simulink model "Simple_4Quad_payload_09_2017a"  (R2018b)
settings: Solver=ode45  StartTime=0.0  StopTime=40  RelTol=1e-3
InitFcn:
  | Simple_4Quad_payload_09_const
values from neighbouring files (symbols this model uses):
  All_rho = [d1 0 0 ... (first row only)    [Colab_4Quad_model_01_const.m]    (also in Colab_4Quad_model_02_const.m; Simple_4Quad_payload_04_const.m; Simple_4Quad_payload_05_const.m; Simple_4Quad_payload_06_const.m)
  alpha_chatt = 0.1    [Simple_4Quad_payload_09_const.m]    (also in Simple_4Quad_payload_10_const.m = 0.001; Simple_4Quad_payload_11_const.m = 0.01; Simple_4Quad_payload_12_const.m = 0.01)
  alphaTF = 0.1    [Simple_4Quad_payload_08_const.m]    (also in Simple_4Quad_payload_09_const.m = 0.5; Simple_4Quad_payload_10_const.m = 1; Simple_4Quad_payload_11_const.m = 0.5; Simple_4Quad_payload_12_const.m = 10)
  B_ob = [zeros(3);eye(3)]    [Simple_4Quad_payload_04_const.m]    (also in Simple_4Quad_payload_05_const.m; Simple_4Quad_payload_06_const.m; Simple_4Quad_payload_07_const.m; Simple_4Quad_payload_08_const.m)
  BBT_inv = ((B'*B)^(-1))*B'    [Simple_2Quad_payload_03_const.m]    (also in Simple_4Quad_payload_04_const.m = ((BR'*BR)^(-1))*BR'; Simple_4Quad_payload_05_const.m = ((BR'*BR)^(-1))*BR'; Simple_4Quad_payload_06_const.m = ((BR'*BR)^(-1))*BR'; Simple_4Quad_payload_07_const.m = ((BR'*BR)^(-1))*BR')
  BR = 1e0*eye(n)    [Simple_4Quad_payload_04_const.m]    (also in Simple_4Quad_payload_05_const.m; Simple_4Quad_payload_06_const.m; Simple_4Quad_payload_07_const.m; Simple_4Quad_payload_08_const.m)
  C_ob = [eye(3) zeros(3)]    [Simple_4Quad_payload_04_const.m]    (also in Simple_4Quad_payload_05_const.m; Simple_4Quad_payload_06_const.m; Simple_4Quad_payload_07_const.m; Simple_4Quad_payload_08_const.m)
  d1 = 0.25    [Colab_4Quad_model_01_const.m]    (also in Colab_4Quad_model_02_const.m = 0.5; Simple_4Quad_payload_01_const.m = 1; Simple_4Quad_payload_02_const.m = 1; Simple_4Quad_payload_03_const.m = 1)
  d2 = 0.25    [Colab_4Quad_model_01_const.m]    (also in Colab_4Quad_model_02_const.m = 0.5; Simple_4Quad_payload_01_const.m = 1; Simple_4Quad_payload_02_const.m = 1; Simple_4Quad_payload_03_const.m = 1)
  Des_rel_dist = 2    [Simple_4Quad_payload_01_const.m]    (also in Simple_4Quad_payload_02_const.m = 4; Simple_4Quad_payload_03_const.m = 4; Simple_4Quad_payload_04_const.m; Simple_4Quad_payload_05_const.m)
  g = 9.81    [Colab_4Quad_model_01_const.m]    (also in Colab_4Quad_model_02_const.m; Simple_2Quad_payload_01_const.m; Simple_2Quad_payload_02_const.m; Simple_2Quad_payload_03_const.m)
  gamma_0 = 1e-0*diag([1e-3;1e-0])    [Simple_2Quad_payload_03_const.m]    (also in Simple_4Quad_payload_04_const.m = 1e-0*diag([1e-6*ones(3,1);1e-0*ones(3,1)]); Simple_4Quad_payload_05_const.m = 1e-1*diag([1e-6*ones(3,1);1e-0*ones(3,1)]); Simple_4Quad_payload_06_const.m = 1e-0*diag([1e-6*ones(3,1);1e-0*ones(3,1)]); Simple_4Quad_payload_07_const.m = 1e-0*diag([1e-6*ones(3,1);1e-0*ones(3,1)]))
  gamma_0L = 1e-0*diag([1e-6*ones(3,1);1e-0*ones(3,1)])    [Simple_4Quad_payload_08_const.m]    (also in Simple_4Quad_payload_09_const.m; Simple_4Quad_payload_10_const.m = 1e+0*diag([1e-3*ones(3,1);1e-3*ones(3,1)]); Simple_4Quad_payload_11_const.m = 1e+0*diag([1e-3*ones(3,1);1e-3*ones(3,1)]); Simple_4Quad_payload_12_const.m = 1e+2*diag(1e-4*ones(3,1)))
  gamma_0v = 1e-0*diag([1e-0*ones(3,1);1e-0*ones(3,1)])    [Simple_4Quad_payload_08_const.m]    (also in Simple_4Quad_payload_09_const.m = 1e-0*diag([1e-6*ones(3,1);1e-6*ones(3,1)]); Simple_4Quad_payload_10_const.m = 1e+0*diag(1e-0*ones(3,1)); Simple_4Quad_payload_11_const.m = 1e+0*diag(1e-0*ones(3,1)); Simple_4Quad_payload_12_const.m = 1e+3*diag(1e-0*ones(3,1)))
  gamma_1 = 1e+2*diag([1e-3;1e-0])    [Simple_2Quad_payload_03_const.m]    (also in Simple_4Quad_payload_04_const.m = 1e+2*diag([1e-6*ones(3,1);1e-0*ones(3,1)]); Simple_4Quad_payload_05_const.m = 1e+2*diag([1e-6*ones(3,1);1e-0*ones(3,1)]); Simple_4Quad_payload_06_const.m = 1e+3*diag([1e-6*ones(3,1);1e-0*ones(3,1)]); Simple_4Quad_payload_07_const.m = 1e+3*diag([1e-6*ones(3,1);1e-0*ones(3,1)]))
  gamma_1L = 1e+3*diag([1e-6*ones(3,1);1e-0*ones(3,1)])    [Simple_4Quad_payload_08_const.m]    (also in Simple_4Quad_payload_09_const.m = 1e+2*diag([1e-6*ones(3,1);1e-0*ones(3,1)]); Simple_4Quad_payload_10_const.m = 1e+1*diag([1e-3*ones(3,1);1e-3*ones(3,1)]); Simple_4Quad_payload_11_const.m = 1e+0*diag([1e-3*ones(3,1);1e-3*ones(3,1)]); Simple_4Quad_payload_12_const.m = 1e+2*diag(1e-4*ones(3,1)))
  gamma_1v = 1e+3*diag([1e-0*ones(3,1);1e-0*ones(3,1)])    [Simple_4Quad_payload_08_const.m]    (also in Simple_4Quad_payload_09_const.m = 1e+2*diag([1e-6*ones(3,1);1e-6*ones(3,1)]); Simple_4Quad_payload_10_const.m = 1e+0*diag(1e-0*ones(3,1)); Simple_4Quad_payload_11_const.m = 1e+0*diag(1e-0*ones(3,1)); Simple_4Quad_payload_12_const.m = 1e+3*diag(1e-0*ones(3,1)))
  Ix = 0.166667    [Colab_4Quad_model_01_const.m]    (also in Colab_4Quad_model_02_const.m = 0.02; Simple_4Quad_payload_01_const.m = 1; Simple_4Quad_payload_02_const.m = 1; Simple_4Quad_payload_03_const.m = 1)
  Iy = 0.166667    [Colab_4Quad_model_01_const.m]    (also in Colab_4Quad_model_02_const.m = 0.02; Simple_4Quad_payload_01_const.m = 1; Simple_4Quad_payload_02_const.m = 1; Simple_4Quad_payload_03_const.m = 1)
  Iz = 0.166667    [Colab_4Quad_model_01_const.m]    (also in Colab_4Quad_model_02_const.m = 0.02; Simple_4Quad_payload_01_const.m = 1; Simple_4Quad_payload_02_const.m = 1; Simple_4Quad_payload_03_const.m = 1)
  Jo = diag([Ix;Iy;Iz])    [Colab_4Quad_model_01_const.m]    (also in Colab_4Quad_model_02_const.m; Simple_4Quad_payload_04_const.m; Simple_4Quad_payload_05_const.m; Simple_4Quad_payload_06_const.m)
  Jq = diag([0.0291 0.0291 0.0552])    [Colab_4Quad_model_01_const.m]    (also in Colab_4Quad_model_02_const.m = diag([0.03 0.03 0.06]); Simple_4Quad_payload_03_const.m = 1.2416e-3 * diag([1 1 2]); Simple_4Quad_payload_04_const.m = 1 * diag([1 1 2]); Simple_4Quad_payload_05_const.m = 1 * diag([1 1 2]))
  k1 = 1    [Simple_2Quad_payload_03_const.m]    (also in Simple_4Quad_payload_04_const.m; Simple_4Quad_payload_05_const.m; Simple_4Quad_payload_06_const.m; Simple_4Quad_payload_07_const.m)
  k2 = 0.1    [Simple_2Quad_payload_03_const.m]    (also in Simple_4Quad_payload_04_const.m; Simple_4Quad_payload_05_const.m; Simple_4Quad_payload_06_const.m; Simple_4Quad_payload_07_const.m)
  l = 3.1819    [Colab_4Quad_model_01_const.m]    (also in Colab_4Quad_model_02_const.m = 3; Simple_2Quad_payload_04_const.m = 1; Simple_4Quad_payload_01_const.m = 1; Simple_4Quad_payload_02_const.m = 2)
  m = 1.5    [Colab_4Quad_model_01_const.m]    (also in Colab_4Quad_model_02_const.m; Simple_2Quad_payload_04_const.m = 1; Simple_4Quad_payload_01_const.m = 1; Simple_4Quad_payload_02_const.m = 1)
  M = 1.0    (= 1)    [Colab_4Quad_model_01_const.m]    (also in Colab_4Quad_model_02_const.m; Simple_2Quad_payload_01_const.m; Simple_2Quad_payload_02_const.m; Simple_2Quad_payload_03_const.m)
  n = 2    [Simple_2Quad_payload_03_const.m]    (also in Simple_4Quad_payload_03_const.m = 6; Simple_4Quad_payload_04_const.m = 6; Simple_4Quad_payload_05_const.m = 6; Simple_4Quad_payload_06_const.m = 6)
  noise_var_Omegao = 0e-6    (= 0)    [Simple_4Quad_payload_07_const.m]    (also in Simple_4Quad_payload_08_const.m; Simple_4Quad_payload_09_const.m; Simple_4Quad_payload_10_const.m; Simple_4Quad_payload_11_const.m)
  noise_var_RelAcc = 0e-6    (= 0)    [Simple_4Quad_payload_07_const.m]    (also in Simple_4Quad_payload_08_const.m; Simple_4Quad_payload_09_const.m; Simple_4Quad_payload_10_const.m; Simple_4Quad_payload_11_const.m)
  noise_var_RelPos = 0e-6    (= 0)    [Simple_4Quad_payload_07_const.m]    (also in Simple_4Quad_payload_08_const.m; Simple_4Quad_payload_09_const.m; Simple_4Quad_payload_10_const.m; Simple_4Quad_payload_11_const.m)
  Q_ob = var_u_ob * eye(6)    [Simple_4Quad_payload_04_const.m]    (also in Simple_4Quad_payload_05_const.m; Simple_4Quad_payload_06_const.m; Simple_4Quad_payload_07_const.m; Simple_4Quad_payload_08_const.m)
  QL = 1e-0*eye(n)    [Simple_4Quad_payload_08_const.m]    (also in Simple_4Quad_payload_09_const.m; Simple_4Quad_payload_10_const.m; Simple_4Quad_payload_11_const.m = 1e-2*eye(n); Simple_4Quad_payload_12_const.m = 1e-0*eye(np))
  QR = 1e-0*eye(n)    [Simple_4Quad_payload_04_const.m]    (also in Simple_4Quad_payload_05_const.m = 1e-1*eye(n); Simple_4Quad_payload_06_const.m; Simple_4Quad_payload_07_const.m; Simple_4Quad_payload_08_const.m)
  Qv = 1e-0*eye(n)    [Simple_4Quad_payload_08_const.m]    (also in Simple_4Quad_payload_09_const.m; Simple_4Quad_payload_10_const.m = 1e-0*eye(np); Simple_4Quad_payload_11_const.m = 1e-2*eye(np); Simple_4Quad_payload_12_const.m = 1e-0*eye(np))
  R = 1e+0*eye(n)    [Simple_2Quad_payload_03_const.m]    (also in Simple_4Quad_payload_04_const.m = 1e+0*eye(m); Simple_4Quad_payload_05_const.m = 1e+0*eye(m); Simple_4Quad_payload_06_const.m; Simple_4Quad_payload_07_const.m)
  R_ob = var_y_ob * eye(3)    [Simple_4Quad_payload_04_const.m]    (also in Simple_4Quad_payload_05_const.m; Simple_4Quad_payload_06_const.m; Simple_4Quad_payload_07_const.m; Simple_4Quad_payload_08_const.m)
  rho_0 = 1e-0    (= 1)    [Simple_2Quad_payload_03_const.m]    (also in Simple_4Quad_payload_04_const.m; Simple_4Quad_payload_05_const.m = 0.1; Simple_4Quad_payload_06_const.m; Simple_4Quad_payload_07_const.m)
  rho_0L = 1e-0    (= 1)    [Simple_4Quad_payload_08_const.m]    (also in Simple_4Quad_payload_09_const.m; Simple_4Quad_payload_10_const.m; Simple_4Quad_payload_11_const.m; Simple_4Quad_payload_12_const.m)
  rho_0v = 1e-1    (= 0.1)    [Simple_4Quad_payload_08_const.m]    (also in Simple_4Quad_payload_09_const.m = 1; Simple_4Quad_payload_10_const.m = 1; Simple_4Quad_payload_11_const.m = 1; Simple_4Quad_payload_12_const.m = 1)
  rho_1 = 1e-0    (= 1)    [Simple_2Quad_payload_03_const.m]    (also in Simple_4Quad_payload_04_const.m; Simple_4Quad_payload_05_const.m; Simple_4Quad_payload_06_const.m; Simple_4Quad_payload_07_const.m)
  rho_1L = 1e-0    (= 1)    [Simple_4Quad_payload_08_const.m]    (also in Simple_4Quad_payload_09_const.m; Simple_4Quad_payload_10_const.m; Simple_4Quad_payload_11_const.m; Simple_4Quad_payload_12_const.m)
  rho_1v = 1e-0    (= 1)    [Simple_4Quad_payload_08_const.m]    (also in Simple_4Quad_payload_09_const.m; Simple_4Quad_payload_10_const.m; Simple_4Quad_payload_11_const.m; Simple_4Quad_payload_12_const.m)
libraries: simulink x1
(part 1 of 4)
settings Model: Creator=ali  LastModifiedBy=asafae
settings SolverCC: ZeroCrossAlgorithm=Adaptive
settings DebuggingCC: IgnoredZcDiagnostic=none
settings CodeAppCC: StateflowObjectComments=on

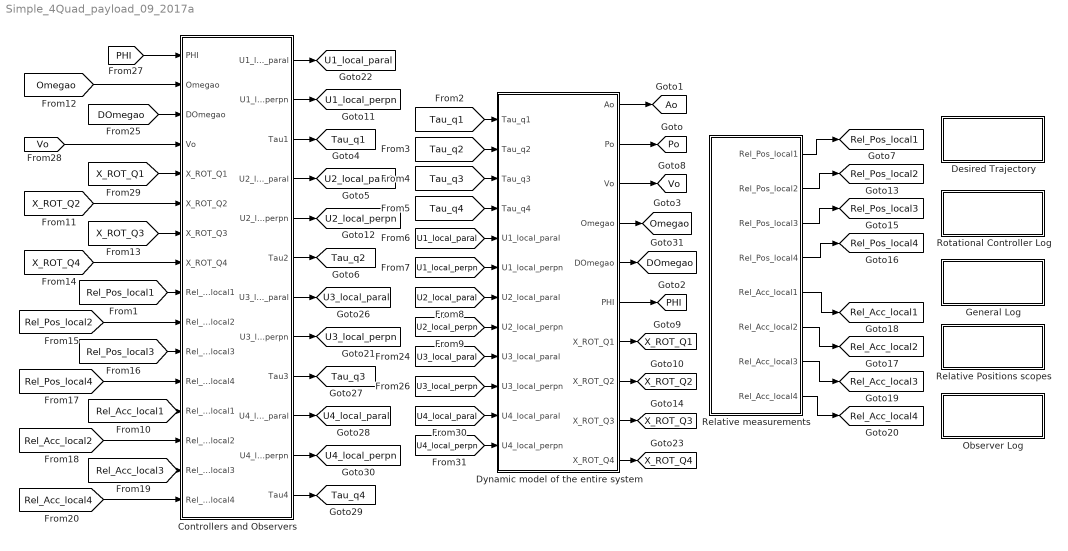
== system Simple_4Quad_payload_09_2017a ==
  Controllers and Observers : Subsystem
  Desired Trajectory : Subsystem
  Dynamic model of the entire system : Subsystem
  General Log : Subsystem
  Observer Log : Subsystem
  Relative Positions scopes : Subsystem
  Relative measurements : Subsystem
  Rotational Controller Log : Subsystem
  tag scope: Ao=global, DOmegao=global, Omegao=global, PHI=global, Po=global, Rel_Acc_local1=global, Rel_Acc_local2=global, Rel_Acc_local3=global, Rel_Acc_local4=global, Rel_Pos_local1=global, Rel_Pos_local2=global, Rel_Pos_local3=global, Rel_Pos_local4=global, Tau_q1=global, Tau_q2=global, Tau_q3=global, Tau_q4=global, U1_local_paral=global, U1_local_perpn=global, U2_local_paral=global, U2_local_perpn=global, U3_local_paral=global, U3_local_perpn=global, U4_local_paral=global, U4_local_perpn=global, Vo=global, X_ROT_Q1=global, X_ROT_Q2=global, X_ROT_Q3=global, X_ROT_Q4=global
  wires:
  [Tau_q1] -> Dynamic model of the entire system/1(Tau_q1)
  [Tau_q2] -> Dynamic model of the entire system/2(Tau_q2)
  [Tau_q3] -> Dynamic model of the entire system/3(Tau_q3)
  [Tau_q4] -> Dynamic model of the entire system/4(Tau_q4)
  [U1_local_paral] -> Dynamic model of the entire system/5(U1_local_paral)
  [U1_local_perpn] -> Dynamic model of the entire system/6(U1_local_perpn)
  Dynamic model of the entire system/6(PHI) -> [PHI]
  Dynamic model of the entire system/4(Omegao) -> [Omegao]
  Dynamic model of the entire system/1(Ao) -> [Ao]
  Dynamic model of the entire system/2(Po) -> [Po]
  Dynamic model of the entire system/5(DOmegao) -> [DOmegao]
  Dynamic model of the entire system/7(X_ROT_Q1) -> [X_ROT_Q1]
  Dynamic model of the entire system/8(X_ROT_Q2) -> [X_ROT_Q2]
  Dynamic model of the entire system/9(X_ROT_Q3) -> [X_ROT_Q3]
  Controllers and Observers/1(U1_local_paral) -> [U1_local_paral]
  Controllers and Observers/3(Tau1) -> [Tau_q1]
  Controllers and Observers/4(U2_local_paral) -> [U2_local_paral]
  Controllers and Observers/6(Tau2) -> [Tau_q2]
  Controllers and Observers/12(Tau4) -> [Tau_q4]
  Controllers and Observers/10(U4_local_paral) -> [U4_local_paral]
  Controllers and Observers/9(Tau3) -> [Tau_q3]
  Controllers and Observers/7(U3_local_paral) -> [U3_local_paral]
  [Omegao] -> Controllers and Observers/2(Omegao)
  [DOmegao] -> Controllers and Observers/3(DOmegao)
  [X_ROT_Q1] -> Controllers and Observers/5(X_ROT_Q1)
  [X_ROT_Q2] -> Controllers and Observers/6(X_ROT_Q2)
  [X_ROT_Q3] -> Controllers and Observers/7(X_ROT_Q3)
  [X_ROT_Q4] -> Controllers and Observers/8(X_ROT_Q4)
  [Rel_Pos_local1] -> Controllers and Observers/9(Rel_Pos_local1)
  [Rel_Pos_local2] -> Controllers and Observers/10(Rel_Pos_local2)
  [Rel_Pos_local3] -> Controllers and Observers/11(Rel_Pos_local3)
  [Rel_Pos_local4] -> Controllers and Observers/12(Rel_Pos_local4)
  [Rel_Acc_local1] -> Controllers and Observers/13(Rel_Acc_local1)
  [Rel_Acc_local2] -> Controllers and Observers/14(Rel_Acc_local2)
  [Rel_Acc_local3] -> Controllers and Observers/15(Rel_Acc_local3)
  [Rel_Acc_local4] -> Controllers and Observers/16(Rel_Acc_local4)
  Relative measurements/1(Rel_Pos_local1) -> [Rel_Pos_local1]
  Relative measurements/2(Rel_Pos_local2) -> [Rel_Pos_local2]
  Relative measurements/3(Rel_Pos_local3) -> [Rel_Pos_local3]
  Relative measurements/4(Rel_Pos_local4) -> [Rel_Pos_local4]
  Relative measurements/5(Rel_Acc_local1) -> [Rel_Acc_local1]
  Relative measurements/6(Rel_Acc_local2) -> [Rel_Acc_local2]
  Relative measurements/7(Rel_Acc_local3) -> [Rel_Acc_local3]
  Relative measurements/8(Rel_Acc_local4) -> [Rel_Acc_local4]
  Dynamic model of the entire system/3(Vo) -> [Vo]
  [Vo] -> Controllers and Observers/4(Vo)
  [PHI] -> Controllers and Observers/1(PHI)
  Controllers and Observers/2(U1_local_perpn) -> [U1_local_perpn]
  Controllers and Observers/5(U2_local_perpn) -> [U2_local_perpn]
  Controllers and Observers/8(U3_local_perpn) -> [U3_local_perpn]
  Controllers and Observers/11(U4_local_perpn) -> [U4_local_perpn]
  [U2_local_paral] -> Dynamic model of the entire system/7(U2_local_paral)
  [U2_local_perpn] -> Dynamic model of the entire system/8(U2_local_perpn)
  [U3_local_paral] -> Dynamic model of the entire system/9(U3_local_paral)
  [U4_local_paral] -> Dynamic model of the entire system/11(U4_local_paral)
  [U4_local_perpn] -> Dynamic model of the entire system/12(U4_local_perpn)
  [U3_local_perpn] -> Dynamic model of the entire system/10(U3_local_perpn)
  Dynamic model of the entire system/10(X_ROT_Q4) -> [X_ROT_Q4]

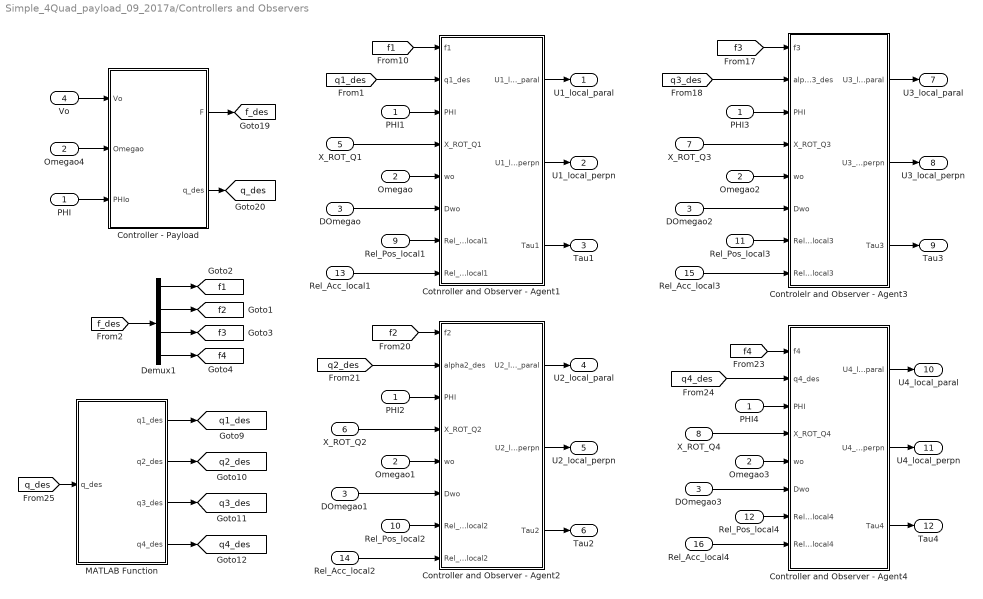
== system Simple_4Quad_payload_09_2017a/Controllers and Observers ==
  PHI : Inport
  Omegao : Inport  Port=2
  DOmegao : Inport  Port=3
  Vo : Inport  Port=4
  X_ROT_Q1 : Inport  Port=5
  X_ROT_Q2 : Inport  Port=6
  X_ROT_Q3 : Inport  Port=7
  X_ROT_Q4 : Inport  Port=8
  Rel_Pos_local1 : Inport  Port=9
  Rel_Pos_local2 : Inport  Port=10
  Rel_Pos_local3 : Inport  Port=11
  Rel_Pos_local4 : Inport  Port=12
  Rel_Acc_local1 : Inport  Port=13
  Rel_Acc_local2 : Inport  Port=14
  Rel_Acc_local3 : Inport  Port=15
  Rel_Acc_local4 : Inport  Port=16
  Controlelr and Observer - Agent3 : Subsystem
  Controller - Payload : Subsystem
  Controller and Observer - Agent2 : Subsystem
  Controller and Observer - Agent4 : Subsystem
  "Cotnroller and Observer - Agent1 " : Subsystem
  DOmegao1 : InportShadow  Port=3
  DOmegao2 : InportShadow  Port=3
  DOmegao3 : InportShadow  Port=3
  Demux1 : Demux
  MATLAB Function : MATLAB Function  TreatAsAtomicUnit=on
  Omegao{1..4} (4 alike) : InportShadow  Port=2
  PHI{1..4} (4 alike) : InportShadow
  U1_local_paral : Outport
  U1_local_perpn : Outport  Port=2
  Tau1 : Outport  Port=3
  U2_local_paral : Outport  Port=4
  U2_local_perpn : Outport  Port=5
  Tau2 : Outport  Port=6
  U3_local_paral : Outport  Port=7
  U3_local_perpn : Outport  Port=8
  Tau3 : Outport  Port=9
  U4_local_paral : Outport  Port=10
  U4_local_perpn : Outport  Port=11
  Tau4 : Outport  Port=12
  tag scope: f1=global, f2=global, f3=global, f4=global, f_des=global, q1_des=global, q2_des=global, q3_des=global, q4_des=global, q_des=global
  wires:
  Controller and Observer - Agent4/3(Tau4) -> Tau4/1
  Controller and Observer - Agent4/1(U4_local_paral) -> U4_local_paral/1
  Controlelr and Observer - Agent3/3(Tau3) -> Tau3/1
  Controlelr and Observer - Agent3/1(U3_local_paral) -> U3_local_paral/1
  Controller and Observer - Agent2/1(U2_local_paral) -> U2_local_paral/1
  "Cotnroller and Observer - Agent1 "/1(U1_local_paral) -> U1_local_paral/1
  Controller and Observer - Agent2/3(Tau2) -> Tau2/1
  X_ROT_Q1/1 -> "Cotnroller and Observer - Agent1 "/4(X_ROT_Q1)
  X_ROT_Q3/1 -> Controlelr and Observer - Agent3/4(X_ROT_Q3)
  X_ROT_Q4/1 -> Controller and Observer - Agent4/4(X_ROT_Q4)
  X_ROT_Q2/1 -> Controller and Observer - Agent2/4(X_ROT_Q2)
  "Cotnroller and Observer - Agent1 "/3(Tau1) -> Tau1/1
  [f1] -> "Cotnroller and Observer - Agent1 "/1(f1)
  Controller - Payload/2(q_des) -> [q_des]
  Vo/1 -> Controller - Payload/1(Vo)
  Omegao4/1 -> Controller - Payload/2(Omegao)
  PHI/1 -> Controller - Payload/3(PHIo)
  Controller - Payload/1(F) -> [f_des]
  Rel_Pos_local1/1 -> "Cotnroller and Observer - Agent1 "/7(Rel_Pos_local1)
  Rel_Acc_local1/1 -> "Cotnroller and Observer - Agent1 "/8(Rel_Acc_local1)
  Rel_Pos_local2/1 -> Controller and Observer - Agent2/7(Rel_Pos_local2)
  Rel_Acc_local2/1 -> Controller and Observer - Agent2/8(Rel_Acc_local2)
  Rel_Pos_local4/1 -> Controller and Observer - Agent4/7(Rel_Pos_local4)
  Rel_Acc_local4/1 -> Controller and Observer - Agent4/8(Rel_Acc_local4)
  Rel_Pos_local3/1 -> Controlelr and Observer - Agent3/7(Rel_Pos_local3)
  Rel_Acc_local3/1 -> Controlelr and Observer - Agent3/8(Rel_Acc_local3)
  [f3] -> Controlelr and Observer - Agent3/1(f3)
  [q3_des] -> Controlelr and Observer - Agent3/2(alpha3_des)
  [f2] -> Controller and Observer - Agent2/1(f2)
  [q2_des] -> Controller and Observer - Agent2/2(alpha2_des)
  [f4] -> Controller and Observer - Agent4/1(f4)
  [q4_des] -> Controller and Observer - Agent4/2(q4_des)
  DOmegao/1 -> "Cotnroller and Observer - Agent1 "/6(Dwo)
  DOmegao1/1 -> Controller and Observer - Agent2/6(Dwo)
  DOmegao2/1 -> Controlelr and Observer - Agent3/6(Dwo)
  DOmegao3/1 -> Controller and Observer - Agent4/6(Dwo)
  Omegao/1 -> "Cotnroller and Observer - Agent1 "/5(wo)
  Omegao2/1 -> Controlelr and Observer - Agent3/5(wo)
  Omegao1/1 -> Controller and Observer - Agent2/5(wo)
  Omegao3/1 -> Controller and Observer - Agent4/5(wo)
  Demux1/4 -> [f4]
  Demux1/1 -> [f1]
  [f_des] -> Demux1/1
  Demux1/3 -> [f3]
  Demux1/2 -> [f2]
  PHI1/1 -> "Cotnroller and Observer - Agent1 "/3(PHI)
  PHI2/1 -> Controller and Observer - Agent2/3(PHI)
  PHI3/1 -> Controlelr and Observer - Agent3/3(PHI)
  PHI4/1 -> Controller and Observer - Agent4/3(PHI)
  [q_des] -> MATLAB Function/1(q_des)
  [q1_des] -> "Cotnroller and Observer - Agent1 "/2(q1_des)
  "Cotnroller and Observer - Agent1 "/2(U1_local_perpn) -> U1_local_perpn/1
  Controller and Observer - Agent2/2(U2_local_perpn) -> U2_local_perpn/1
  Controlelr and Observer - Agent3/2(U3_local_perpn) -> U3_local_perpn/1
  Controller and Observer - Agent4/2(U4_local_perpn) -> U4_local_perpn/1
  MATLAB Function/4(q4_des) -> [q4_des]
  MATLAB Function/3(q3_des) -> [q3_des]
  MATLAB Function/2(q2_des) -> [q2_des]
  MATLAB Function/1(q1_des) -> [q1_des]

== system Simple_4Quad_payload_09_2017a/Desired Trajectory ==
  Clock : Clock
  Constant1 : Constant  Value=[0;0;0]
  Constant2 : Constant  Value=[0;0;2]
  Constant3 : Constant  Value=[0.3;0.5;2]
  Gain : Gain  Gain=0.01
  Gain1 : Gain  Gain=0.02
  MATLAB Function : MATLAB Function  TreatAsAtomicUnit=on
  Mux3 : Mux  Inputs=3
  Subsystem : Subsystem
  Switch : Switch  Criteria=u2 > Threshold  Threshold=10
  Switch1 : Switch  Criteria=u2 > Threshold  Threshold=20
  tag scope: Desired_Track=global
  wires:
  Constant3/1 -> Switch1/1
  Gain/1 -> Mux3/1
  Constant1/1 -> Switch/3
  Gain1/1 -> Mux3/2
  Switch/1 -> Switch1/3
  Constant2/1 -> Switch/1
  Switch1/1 -> Subsystem/1(In1)
  Clock/1 -> Gain1/1, Switch1/2, Switch/2, MATLAB Function/1(t), Gain/1
  Subsystem/1(Out1) -> [Desired_Track]

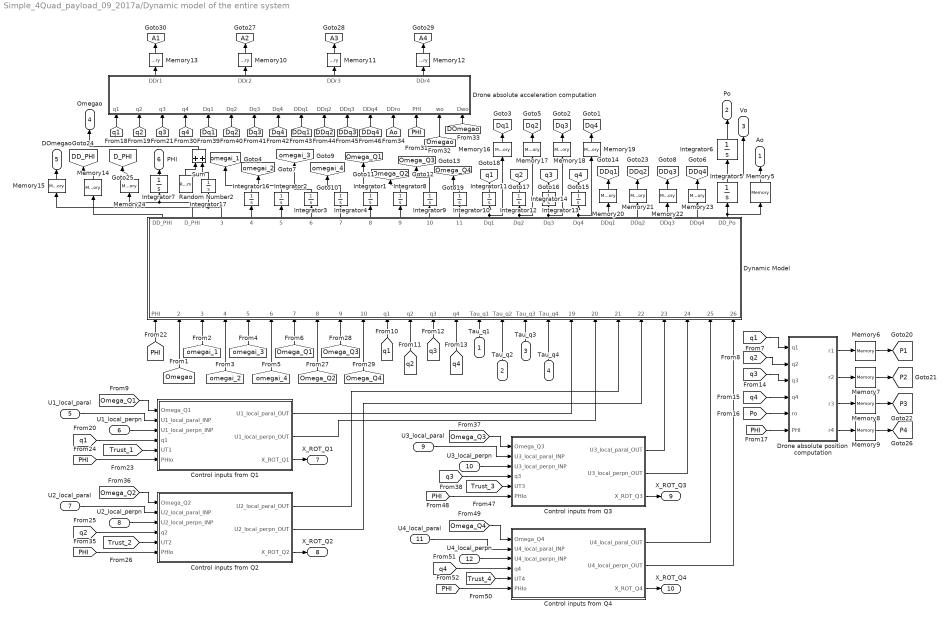
== system Simple_4Quad_payload_09_2017a/Dynamic model of the entire system ==
  Tau_q1 : Inport
  Tau_q2 : Inport  Port=2
  Tau_q3 : Inport  Port=3
  Tau_q4 : Inport  Port=4
  U1_local_paral : Inport  Port=5
  U1_local_perpn : Inport  Port=6
  U2_local_paral : Inport  Port=7
  U2_local_perpn : Inport  Port=8
  U3_local_paral : Inport  Port=9
  U3_local_perpn : Inport  Port=10
  U4_local_paral : Inport  Port=11
  U4_local_perpn : Inport  Port=12
  Control inputs from Q1 : Subsystem
  Control inputs from Q2 : Subsystem
  Control inputs from Q3 : Subsystem
  Control inputs from Q4 : Subsystem
  Drone absolute acceleration computation : MATLAB Function  TreatAsAtomicUnit=on
  Drone absolute position computation : MATLAB Function  TreatAsAtomicUnit=on
  "Dynamic Model " : MATLAB Function  TreatAsAtomicUnit=on
  Integrator{1..5,7..10,16..17} (11 alike) : Integrator  InitialCondition=zeros(3,1)
  Integrator{11..14} (4 alike) : Integrator  InitialCondition=[0;0;1]
  Integrator6 : Integrator  InitialCondition=[0;0;0]
  Memory{5,10..24} (16 alike) : Memory  InitialCondition=zeros(3,1)
  Memory6 : Memory  InitialCondition=[d1;0;l]
  Memory7 : Memory  InitialCondition=[-d1;0;l]
  Memory8 : Memory  InitialCondition=[0;d2;l]
  Memory9 : Memory  InitialCondition=[0;-d2;l]
  Random Number2 : RandomNumber  Variance=noise_var_Omegao  VectorParams1D=off
  Sum : Sum
  Ao : Outport
  Po : Outport  Port=2
  Vo : Outport  Port=3
  Omegao : Outport  Port=4
  DOmegao : Outport  Port=5
  PHI : Outport  Port=6
  X_ROT_Q1 : Outport  Port=7
  X_ROT_Q2 : Outport  Port=8
  X_ROT_Q3 : Outport  Port=9
  X_ROT_Q4 : Outport  Port=10
  tag scope: A1=global, A2=global, A3=global, A4=global, DD_PHI=global, DDq1=global, DDq2=global, DDq3=global, DDq4=global, D_PHI=global, Dq1=global, Dq2=global, Dq3=global, Dq4=global, Omega_Q1=global, Omega_Q2=global, Omega_Q3=global, Omega_Q4=global, P1=global, P2=global, P3=global, P4=global, omegai_1=global, omegai_2=global, omegai_3=global, omegai_4=global, q1=global, q2=global, q3=global, q4=global
  wires:
  Integrator5/1 -> Vo/1, Integrator6/1
  Integrator1/1 -> [Omega_Q1]
  Integrator2/1 -> [omegai_2]
  Integrator3/1 -> [omegai_3]
  Integrator6/1 -> Po/1
  Integrator4/1 -> [omegai_4]
  Memory5/1 -> Ao/1
  Integrator7/1 -> PHI/1
  "Dynamic Model "/20(DD_Po) -> Memory5/1, Integrator5/1
  "Dynamic Model "/2(D_PHI) -> Memory24/1, Integrator7/1
  "Dynamic Model "/1(DD_PHI) -> Memory14/1
  "Dynamic Model "/7(D_omegai_4) -> Integrator4/1
  "Dynamic Model "/6(D_omegai_3) -> Integrator3/1
  "Dynamic Model "/5(D_omegai_2) -> Integrator2/1
  "Dynamic Model "/4(D_omegai_1) -> Integrator16/1
  "Dynamic Model "/3(D_Omegao) -> Memory15/1, Integrator17/1
  Integrator16/1 -> [omegai_1]
  "Dynamic Model "/8(D_Omega_Q1) -> Integrator1/1
  "Dynamic Model "/9(D_Omega_Q2) -> Integrator8/1
  "Dynamic Model "/10(D_Omega_Q3) -> Integrator9/1
  "Dynamic Model "/11(D_Omega_Q4) -> Integrator10/1
  Integrator8/1 -> [Omega_Q2]
  Integrator10/1 -> [Omega_Q4]
  Integrator9/1 -> [Omega_Q3]
  "Dynamic Model "/12(Dq1) -> Memory16/1, Integrator11/1
  "Dynamic Model "/13(Dq2) -> Memory17/1, Integrator12/1
  "Dynamic Model "/14(Dq3) -> Memory18/1, Integrator13/1
  "Dynamic Model "/15(Dq4) -> Memory19/1, Integrator14/1
  Integrator14/1 -> [q4]
  Integrator13/1 -> [q3]
  Integrator12/1 -> [q2]
  Integrator11/1 -> [q1]
  [PHI] -> "Dynamic Model "/1(PHI)
  [Omegao] -> "Dynamic Model "/2(Omegao)
  [omegai_1] -> "Dynamic Model "/3(omegai1)
  [omegai_2] -> "Dynamic Model "/4(omegai2)
  [omegai_3] -> "Dynamic Model "/5(omegai3)
  [omegai_4] -> "Dynamic Model "/6(omegai4)
  [Omega_Q1] -> "Dynamic Model "/7(Omega_q1)
  [Omega_Q2] -> "Dynamic Model "/8(Omega_q2)
  [Omega_Q3] -> "Dynamic Model "/9(Omega_q3)
  [Omega_Q4] -> "Dynamic Model "/10(Omega_q4)
  [q1] -> "Dynamic Model "/11(q1)
  [q2] -> "Dynamic Model "/12(q2)
  [q3] -> "Dynamic Model "/13(q3)
  [q4] -> "Dynamic Model "/14(q4)
  Tau_q2/1 -> "Dynamic Model "/16(Tau_q2)
  Tau_q4/1 -> "Dynamic Model "/18(Tau_q4)
  Tau_q1/1 -> "Dynamic Model "/15(Tau_q1)
  Tau_q3/1 -> "Dynamic Model "/17(Tau_q3)
  Control inputs from Q1/1(U1_local_paral_OUT) -> "Dynamic Model "/19(U1_local_paral)
  [q1] -> Drone absolute position computation/1(q1)
  [q2] -> Drone absolute position computation/2(q2)
  [q3] -> Drone absolute position computation/3(q3)
  [q4] -> Drone absolute position computation/4(q4)
  [Po] -> Drone absolute position computation/5(ro)
  [PHI] -> Drone absolute position computation/6(PHI)
  Memory6/1 -> [P1]
  Memory8/1 -> [P3]
  Memory7/1 -> [P2]
  Memory9/1 -> [P4]
  Drone absolute position computation/4(r4) -> Memory9/1
  Drone absolute position computation/3(r3) -> Memory8/1
  Drone absolute position computation/2(r2) -> Memory7/1
  Drone absolute position computation/1(r1) -> Memory6/1
  [q1] -> Drone absolute acceleration computation/1(q1)
  [q2] -> Drone absolute acceleration computation/2(q2)
  [q3] -> Drone absolute acceleration computation/3(q3)
  [q4] -> Drone absolute acceleration computation/4(q4)
  [PHI] -> Drone absolute acceleration computation/14(PHI)
  [Omegao] -> Drone absolute acceleration computation/15(wo)
  Memory13/1 -> [A1]
  Drone absolute acceleration computation/1(DDr1) -> Memory13/1
  Memory10/1 -> [A2]
  Drone absolute acceleration computation/2(DDr2) -> Memory10/1
  Memory11/1 -> [A3]
  Drone absolute acceleration computation/3(DDr3) -> Memory11/1
  Memory12/1 -> [A4]
  Drone absolute acceleration computation/4(DDr4) -> Memory12/1
  Memory15/1 -> DOmegao/1
  [DOmegao] -> Drone absolute acceleration computation/16(Dwo)
  [Ao] -> Drone absolute acceleration computation/13(DDro)
  Memory19/1 -> [Dq4]
  Memory18/1 -> [Dq3]
  Memory16/1 -> [Dq1]
  Memory17/1 -> [Dq2]
  [Dq4] -> Drone absolute acceleration computation/8(Dq4)
  [Dq3] -> Drone absolute acceleration computation/7(Dq3)
  [Dq2] -> Drone absolute acceleration computation/6(Dq2)
  [Dq1] -> Drone absolute acceleration computation/5(Dq1)
  Memory21/1 -> [DDq2]
  Memory20/1 -> [DDq1]
  Memory22/1 -> [DDq3]
  Memory23/1 -> [DDq4]
  "Dynamic Model "/16(DDq1) -> Memory20/1
  "Dynamic Model "/17(DDq2) -> Memory21/1
  "Dynamic Model "/18(DDq3) -> Memory22/1
  "Dynamic Model "/19(DDq4) -> Memory23/1
  [DDq1] -> Drone absolute acceleration computation/9(DDq1)
  [DDq2] -> Drone absolute acceleration computation/10(DDq2)
  [DDq3] -> Drone absolute acceleration computation/11(DDq3)
  [DDq4] -> Drone absolute acceleration computation/12(DDq4)
  Memory24/1 -> [D_PHI]
  Control inputs from Q3/1(U3_local_paral_OUT) -> "Dynamic Model "/23(U3_local_paral)
  Control inputs from Q4/1(U4_local_paral_OUT) -> "Dynamic Model "/25(U4_local_paral)
  Control inputs from Q4/2(U4_local_perpn_OUT) -> "Dynamic Model "/26(U4_local_perpn)
  Control inputs from Q1/3(X_ROT_Q1) -> X_ROT_Q1/1
  [Omega_Q1] -> Control inputs from Q1/1(Omega_Q1)
  U1_local_paral/1 -> Control inputs from Q1/2(U1_local_paral_INP)
  U1_local_perpn/1 -> Control inputs from Q1/3(U1_local_perpn_INP)
  Control inputs from Q1/2(U1_local_perpn_OUT) -> "Dynamic Model "/20(U1_local_perpn)
  [q1] -> Control inputs from Q1/4(q1)
  [Trust_1] -> Control inputs from Q1/5(UT1)
  [PHI] -> Control inputs from Q1/6(PHIo)
  [PHI] -> Control inputs from Q2/6(PHIo)
  [Trust_2] -> Control inputs from Q2/5(UT2)
  [q2] -> Control inputs from Q2/4(q2)
  U2_local_perpn/1 -> Control inputs from Q2/3(U2_local_perpn_INP)
  U2_local_paral/1 -> Control inputs from Q2/2(U2_local_paral_INP)
  [Omega_Q2] -> Control inputs from Q2/1(Omega_Q2)
  Control inputs from Q2/3(X_ROT_Q2) -> X_ROT_Q2/1
  Control inputs from Q2/1(U2_local_paral_OUT) -> "Dynamic Model "/21(U2_local_paral)
  Control inputs from Q2/2(U2_local_perpn_OUT) -> "Dynamic Model "/22(U2_local_perpn)
  [Omega_Q3] -> Control inputs from Q3/1(Omega_Q3)
  U3_local_paral/1 -> Control inputs from Q3/2(U3_local_paral_INP)
  U3_local_perpn/1 -> Control inputs from Q3/3(U3_local_perpn_INP)
  Control inputs from Q3/3(X_ROT_Q3) -> X_ROT_Q3/1
  Control inputs from Q3/2(U3_local_perpn_OUT) -> "Dynamic Model "/24(U3_local_perpn)
  [q3] -> Control inputs from Q3/4(q3)
  [Trust_3] -> Control inputs from Q3/5(UT3)
  [PHI] -> Control inputs from Q3/6(PHIo)
  Control inputs from Q4/3(X_ROT_Q4) -> X_ROT_Q4/1
  U4_local_perpn/1 -> Control inputs from Q4/3(U4_local_perpn_INP)
  U4_local_paral/1 -> Control inputs from Q4/2(U4_local_paral_INP)
  [Omega_Q4] -> Control inputs from Q4/1(Omega_Q4)
  [q4] -> Control inputs from Q4/4(q4)
  [PHI] -> Control inputs from Q4/6(PHIo)
  Memory14/1 -> [DD_PHI]
  [Trust_4] -> Control inputs from Q4/5(UT4)
  Sum/1 -> Omegao/1
  Integrator17/1 -> Sum/2
  Random Number2/1 -> Sum/1

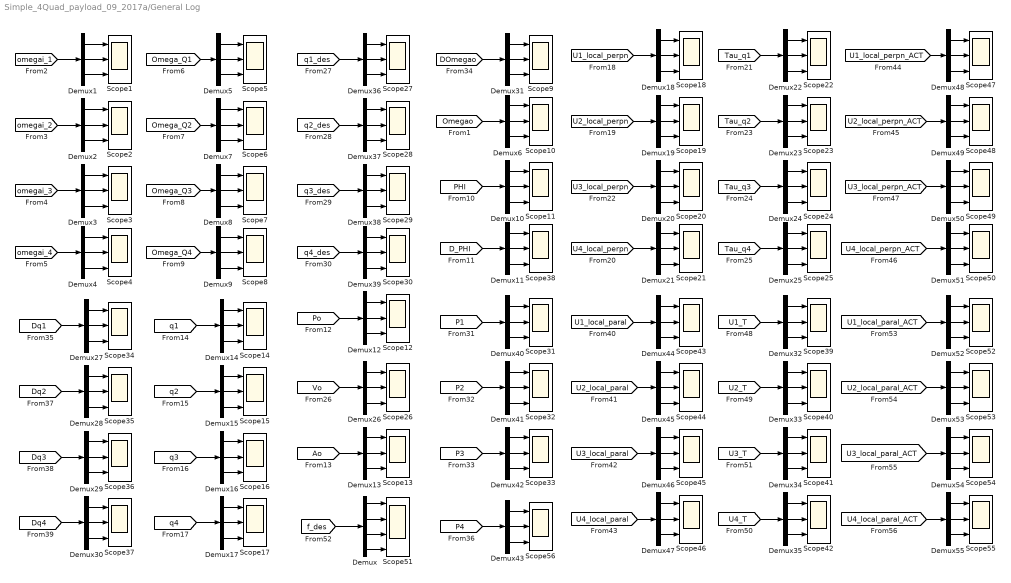
== system Simple_4Quad_payload_09_2017a/General Log ==
  Demux : Demux
  Demux{1..55} (55 alike) : Demux  Outputs=3
  Scope{1..50,52..56} (55 alike) : Scope  NumInputPorts=3
  Scope51 : Scope  NumInputPorts=4
  wires:
  Demux6/2 -> Scope10/2
  Demux6/1 -> Scope10/1
  Demux6/3 -> Scope10/3
  [Omegao] -> Demux6/1
  [omegai_1] -> Demux1/1
  Demux1/3 -> Scope1/3
  Demux1/1 -> Scope1/1
  Demux1/2 -> Scope1/2
  Demux2/2 -> Scope2/2
  Demux2/1 -> Scope2/1
  Demux2/3 -> Scope2/3
  [omegai_2] -> Demux2/1
  [omegai_3] -> Demux3/1
  Demux3/3 -> Scope3/3
  Demux3/1 -> Scope3/1
  Demux3/2 -> Scope3/2
  Demux4/2 -> Scope4/2
  Demux4/1 -> Scope4/1
  Demux4/3 -> Scope4/3
  [omegai_4] -> Demux4/1
  [Omega_Q4] -> Demux9/1
  Demux9/3 -> Scope8/3
  Demux9/1 -> Scope8/1
  Demux9/2 -> Scope8/2
  Demux8/2 -> Scope7/2
  Demux8/1 -> Scope7/1
  Demux8/3 -> Scope7/3
  [Omega_Q3] -> Demux8/1
  [Omega_Q2] -> Demux7/1
  Demux7/3 -> Scope6/3
  Demux7/1 -> Scope6/1
  Demux7/2 -> Scope6/2
  Demux5/2 -> Scope5/2
  Demux5/1 -> Scope5/1
  Demux5/3 -> Scope5/3
  [Omega_Q1] -> Demux5/1
  [PHI] -> Demux10/1
  Demux10/3 -> Scope11/3
  Demux10/1 -> Scope11/1
  Demux10/2 -> Scope11/2
  Demux11/2 -> Scope38/2
  Demux11/1 -> Scope38/1
  Demux11/3 -> Scope38/3
  [D_PHI] -> Demux11/1
  [Po] -> Demux12/1
  Demux12/3 -> Scope12/3
  Demux12/1 -> Scope12/1
  Demux12/2 -> Scope12/2
  Demux13/2 -> Scope13/2
  Demux13/1 -> Scope13/1
  Demux13/3 -> Scope13/3
  [Ao] -> Demux13/1
  [q4] -> Demux17/1
  Demux17/3 -> Scope17/3
  Demux17/1 -> Scope17/1
  Demux17/2 -> Scope17/2
  Demux16/2 -> Scope16/2
  Demux16/1 -> Scope16/1
  Demux16/3 -> Scope16/3
  [q3] -> Demux16/1
  [q2] -> Demux15/1
  Demux15/3 -> Scope15/3
  Demux15/1 -> Scope15/1
  Demux15/2 -> Scope15/2
  Demux14/2 -> Scope14/2
  Demux14/1 -> Scope14/1
  Demux14/3 -> Scope14/3
  [q1] -> Demux14/1
  [U1_local_perpn] -> Demux18/1
  Demux18/3 -> Scope18/3
  Demux18/1 -> Scope18/1
  Demux18/2 -> Scope18/2
  Demux19/2 -> Scope19/2
  Demux19/1 -> Scope19/1
  Demux19/3 -> Scope19/3
  [U2_local_perpn] -> Demux19/1
  [U3_local_perpn] -> Demux20/1
  Demux20/3 -> Scope20/3
  Demux20/1 -> Scope20/1
  Demux20/2 -> Scope20/2
  Demux21/2 -> Scope21/2
  Demux21/1 -> Scope21/1
  Demux21/3 -> Scope21/3
  [U4_local_perpn] -> Demux21/1
  [Tau_q4] -> Demux25/1
  Demux25/3 -> Scope25/3
  Demux25/1 -> Scope25/1
  Demux25/2 -> Scope25/2
  Demux24/2 -> Scope24/2
  Demux24/1 -> Scope24/1
  Demux24/3 -> Scope24/3
  [Tau_q3] -> Demux24/1
  [Tau_q2] -> Demux23/1
  Demux23/3 -> Scope23/3
  Demux23/1 -> Scope23/1
  Demux23/2 -> Scope23/2
  Demux22/2 -> Scope22/2
  Demux22/1 -> Scope22/1
  Demux22/3 -> Scope22/3
  [Tau_q1] -> Demux22/1
  [Vo] -> Demux26/1
  Demux26/3 -> Scope26/3
  Demux26/1 -> Scope26/1
  Demux26/2 -> Scope26/2
  [DOmegao] -> Demux31/1
  Demux31/3 -> Scope9/3
  Demux31/1 -> Scope9/1
  Demux31/2 -> Scope9/2
  [Dq1] -> Demux27/1
  Demux27/3 -> Scope34/3
  Demux27/1 -> Scope34/1
  Demux27/2 -> Scope34/2
  Demux28/2 -> Scope35/2
  Demux28/1 -> Scope35/1
  Demux28/3 -> Scope35/3
  [Dq2] -> Demux28/1
  [Dq3] -> Demux29/1
  Demux29/3 -> Scope36/3
  Demux29/1 -> Scope36/1
  Demux29/2 -> Scope36/2
  Demux30/2 -> Scope37/2
  Demux30/1 -> Scope37/1
  Demux30/3 -> Scope37/3
  [Dq4] -> Demux30/1
  [U4_T] -> Demux35/1
  Demux35/3 -> Scope42/3
  Demux35/1 -> Scope42/1
  Demux35/2 -> Scope42/2
  Demux34/2 -> Scope41/2
  Demux34/1 -> Scope41/1
  Demux34/3 -> Scope41/3
  [U3_T] -> Demux34/1
  [U2_T] -> Demux33/1
  Demux33/3 -> Scope40/3
  Demux33/1 -> Scope40/1
  Demux33/2 -> Scope40/2
  Demux32/2 -> Scope39/2
  Demux32/1 -> Scope39/1
  Demux32/3 -> Scope39/3
  [U1_T] -> Demux32/1
  Demux/1 -> Scope51/1
  Demux/3 -> Scope51/3
  Demux/2 -> Scope51/2
  Demux/4 -> Scope51/4
  [f_des] -> Demux/1
  [q1_des] -> Demux36/1
  Demux36/3 -> Scope27/3
  Demux36/1 -> Scope27/1
  Demux36/2 -> Scope27/2
  Demux37/2 -> Scope28/2
  Demux37/1 -> Scope28/1
  Demux37/3 -> Scope28/3
  [q2_des] -> Demux37/1
  [q3_des] -> Demux38/1
  Demux38/3 -> Scope29/3
  Demux38/1 -> Scope29/1
  Demux38/2 -> Scope29/2
  Demux39/2 -> Scope30/2
  Demux39/1 -> Scope30/1
  Demux39/3 -> Scope30/3
  [q4_des] -> Demux39/1
  [P1] -> Demux40/1
  Demux40/3 -> Scope31/3
  Demux40/2 -> Scope31/2
  Demux41/2 -> Scope32/2
  Demux41/1 -> Scope32/1
  Demux41/3 -> Scope32/3
  [P2] -> Demux41/1
  [P3] -> Demux42/1
  Demux42/3 -> Scope33/3
  Demux42/1 -> Scope33/1
  Demux42/2 -> Scope33/2
  Demux43/2 -> Scope56/2
  Demux43/1 -> Scope56/1
  Demux43/3 -> Scope56/3
  [P4] -> Demux43/1
  Demux40/1 -> Scope31/1
  Demux47/3 -> Scope46/3
  Demux47/1 -> Scope46/1
  Demux47/2 -> Scope46/2
  Demux46/2 -> Scope45/2
  Demux46/1 -> Scope45/1
  Demux46/3 -> Scope45/3
  Demux45/3 -> Scope44/3
  Demux45/1 -> Scope44/1
  Demux45/2 -> Scope44/2
  Demux44/2 -> Scope43/2
  Demux44/1 -> Scope43/1
  Demux44/3 -> Scope43/3
  [U1_local_paral] -> Demux44/1
  [U4_local_paral] -> Demux47/1
  [U3_local_paral] -> Demux46/1
  [U2_local_paral] -> Demux45/1
  [U2_local_paral_ACT] -> Demux53/1
  [U3_local_paral_ACT] -> Demux54/1
  [U4_local_paral_ACT] -> Demux55/1
  [U1_local_paral_ACT] -> Demux52/1
  Demux52/3 -> Scope52/3
  Demux52/1 -> Scope52/1
  Demux52/2 -> Scope52/2
  Demux53/2 -> Scope53/2
  Demux53/1 -> Scope53/1
  Demux53/3 -> Scope53/3
  Demux54/3 -> Scope54/3
  Demux54/1 -> Scope54/1
  Demux54/2 -> Scope54/2
  Demux55/2 -> Scope55/2
  Demux55/1 -> Scope55/1
  Demux55/3 -> Scope55/3
  [U4_local_perpn_ACT] -> Demux51/1
  Demux51/3 -> Scope50/3
  Demux51/1 -> Scope50/1
  Demux51/2 -> Scope50/2
  Demux50/2 -> Scope49/2
  Demux50/1 -> Scope49/1
  Demux50/3 -> Scope49/3
  [U3_local_perpn_ACT] -> Demux50/1
  [U2_local_perpn_ACT] -> Demux49/1
  Demux49/3 -> Scope48/3
  Demux49/1 -> Scope48/1
  Demux49/2 -> Scope48/2
  Demux48/2 -> Scope47/2
  Demux48/1 -> Scope47/1
  Demux48/3 -> Scope47/3
  [U1_local_perpn_ACT] -> Demux48/1

== system Simple_4Quad_payload_09_2017a/Observer Log ==
  Scope{,1..3,8..11} (8 alike) : Scope
  wires:
  [q1_hat] -> Scope/1
  [q2_hat] -> Scope1/1
  [q3_hat] -> Scope2/1
  [q4_hat] -> Scope3/1
  [Dq4_hat] -> Scope11/1
  [Dq3_hat] -> Scope10/1
  [Dq2_hat] -> Scope9/1
  [Dq1_hat] -> Scope8/1

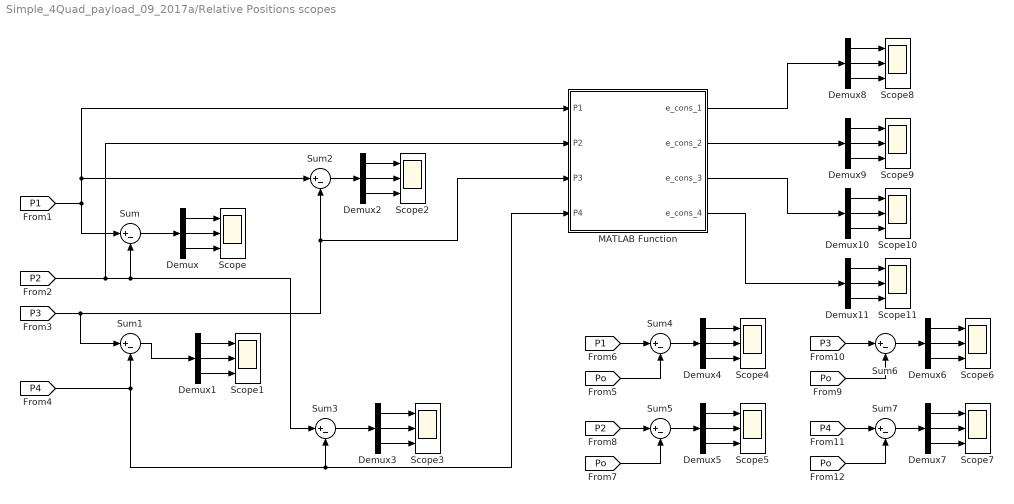
== system Simple_4Quad_payload_09_2017a/Relative Positions scopes ==
  Demux{,1..11} (12 alike) : Demux  Outputs=3
  MATLAB Function : MATLAB Function  TreatAsAtomicUnit=on
  Scope{,1..11} (12 alike) : Scope  NumInputPorts=3
  Sum{,1..7} (8 alike) : Sum  Inputs=|+-
  wires:
  Demux/3 -> Scope/3
  Demux/1 -> Scope/1
  Demux/2 -> Scope/2
  Sum/1 -> Demux/1
  Sum1/1 -> Demux1/1
  Demux1/2 -> Scope1/2
  Demux1/1 -> Scope1/1
  Demux1/3 -> Scope1/3
  Sum2/1 -> Demux2/1
  [P3] -> MATLAB Function/3(P3), Sum2/2, Sum1/1
  [P1] -> Sum/1, Sum2/1, MATLAB Function/1(P1)
  Demux2/2 -> Scope2/2
  Demux2/1 -> Scope2/1
  Demux2/3 -> Scope2/3
  Demux3/3 -> Scope3/3
  Demux3/1 -> Scope3/1
  Demux3/2 -> Scope3/2
  [P2] -> MATLAB Function/2(P2), Sum/2, Sum3/1
  [P4] -> Sum3/2, MATLAB Function/4(P4), Sum1/2
  Sum3/1 -> Demux3/1
  Demux4/3 -> Scope4/3
  Demux4/1 -> Scope4/1
  Demux4/2 -> Scope4/2
  Sum4/1 -> Demux4/1
  Sum5/1 -> Demux5/1
  Demux5/2 -> Scope5/2
  Demux5/1 -> Scope5/1
  Demux5/3 -> Scope5/3
  Demux6/3 -> Scope6/3
  Demux6/1 -> Scope6/1
  Demux6/2 -> Scope6/2
  Sum6/1 -> Demux6/1
  Sum7/1 -> Demux7/1
  Demux7/2 -> Scope7/2
  Demux7/1 -> Scope7/1
  Demux7/3 -> Scope7/3
  [Po] -> Sum4/2
  [P1] -> Sum4/1
  [P2] -> Sum5/1
  [Po] -> Sum5/2
  [P3] -> Sum6/1
  [Po] -> Sum6/2
  [P4] -> Sum7/1
  [Po] -> Sum7/2
  Demux8/2 -> Scope8/2
  Demux8/1 -> Scope8/1
  Demux8/3 -> Scope8/3
  MATLAB Function/1(e_cons_1) -> Demux8/1
  Demux9/3 -> Scope9/3
  Demux9/1 -> Scope9/1
  Demux9/2 -> Scope9/2
  MATLAB Function/2(e_cons_2) -> Demux9/1
  Demux10/2 -> Scope10/2
  Demux10/1 -> Scope10/1
  Demux10/3 -> Scope10/3
  MATLAB Function/3(e_cons_3) -> Demux10/1
  Demux11/3 -> Scope11/3
  Demux11/1 -> Scope11/1
  Demux11/2 -> Scope11/2
  MATLAB Function/4(e_cons_4) -> Demux11/1

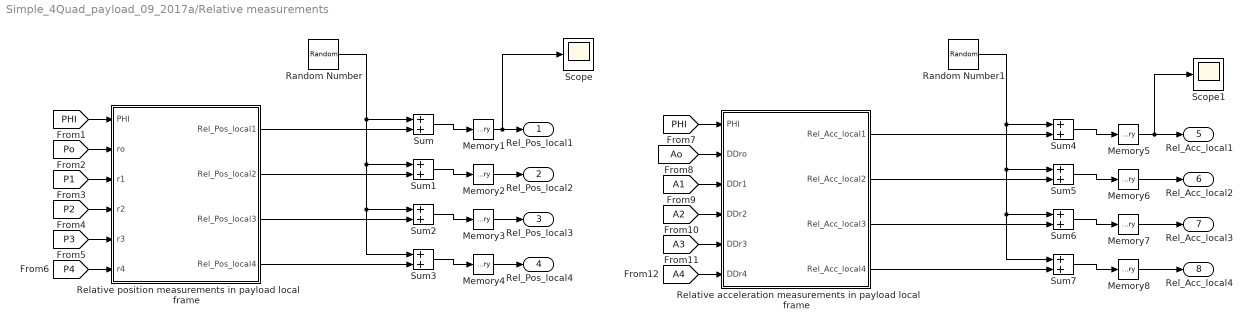
== system Simple_4Quad_payload_09_2017a/Relative measurements ==
  Memory{1..8} (8 alike) : Memory  InitialCondition=zeros(3,1)
  Random Number : RandomNumber  Variance=noise_var_RelPos  VectorParams1D=off
  Random Number1 : RandomNumber  Variance=noise_var_RelAcc  VectorParams1D=off
  Relative acceleration measurements in payload local frame : MATLAB Function  TreatAsAtomicUnit=on
  Relative position measurements in payload local frame : MATLAB Function  TreatAsAtomicUnit=on
  Scope : Scope
  Scope1 : Scope
  Sum{,1..7} (8 alike) : Sum
  Rel_Pos_local1 : Outport
  Rel_Pos_local2 : Outport  Port=2
  Rel_Pos_local3 : Outport  Port=3
  Rel_Pos_local4 : Outport  Port=4
  Rel_Acc_local1 : Outport  Port=5
  Rel_Acc_local2 : Outport  Port=6
  Rel_Acc_local3 : Outport  Port=7
  Rel_Acc_local4 : Outport  Port=8
  wires:
  [PHI] -> Relative position measurements in payload local frame/1(PHI)
  [Po] -> Relative position measurements in payload local frame/2(ro)
  [P1] -> Relative position measurements in payload local frame/3(r1)
  [P2] -> Relative position measurements in payload local frame/4(r2)
  [P3] -> Relative position measurements in payload local frame/5(r3)
  [P4] -> Relative position measurements in payload local frame/6(r4)
  Sum/1 -> Memory1/1
  Sum1/1 -> Memory2/1
  Sum4/1 -> Memory5/1
  [A4] -> Relative acceleration measurements in payload local frame/6(DDr4)
  [A3] -> Relative acceleration measurements in payload local frame/5(DDr3)
  [A2] -> Relative acceleration measurements in payload local frame/4(DDr2)
  [A1] -> Relative acceleration measurements in payload local frame/3(DDr1)
  [Ao] -> Relative acceleration measurements in payload local frame/2(DDro)
  [PHI] -> Relative acceleration measurements in payload local frame/1(PHI)
  Memory1/1 -> Scope/1, Rel_Pos_local1/1
  Memory2/1 -> Rel_Pos_local2/1
  Memory3/1 -> Rel_Pos_local3/1
  Memory4/1 -> Rel_Pos_local4/1
  Memory5/1 -> Scope1/1, Rel_Acc_local1/1
  Memory6/1 -> Rel_Acc_local2/1
  Memory7/1 -> Rel_Acc_local3/1
  Memory8/1 -> Rel_Acc_local4/1
  Relative position measurements in payload local frame/1(Rel_Pos_local1) -> Sum/2
  Relative position measurements in payload local frame/2(Rel_Pos_local2) -> Sum1/2
  Sum2/1 -> Memory3/1
  Relative position measurements in payload local frame/3(Rel_Pos_local3) -> Sum2/2
  Sum3/1 -> Memory4/1
  Relative position measurements in payload local frame/4(Rel_Pos_local4) -> Sum3/2
  Relative acceleration measurements in payload local frame/1(Rel_Acc_local1) -> Sum4/2
  Sum5/1 -> Memory6/1
  Relative acceleration measurements in payload local frame/2(Rel_Acc_local2) -> Sum5/2
  Sum6/1 -> Memory7/1
  Relative acceleration measurements in payload local frame/3(Rel_Acc_local3) -> Sum6/2
  Sum7/1 -> Memory8/1
  Relative acceleration measurements in payload local frame/4(Rel_Acc_local4) -> Sum7/2
  Random Number/1 -> Sum3/1, Sum2/1, Sum1/1, Sum/1
  Random Number1/1 -> Sum7/1, Sum6/1, Sum5/1, Sum4/1

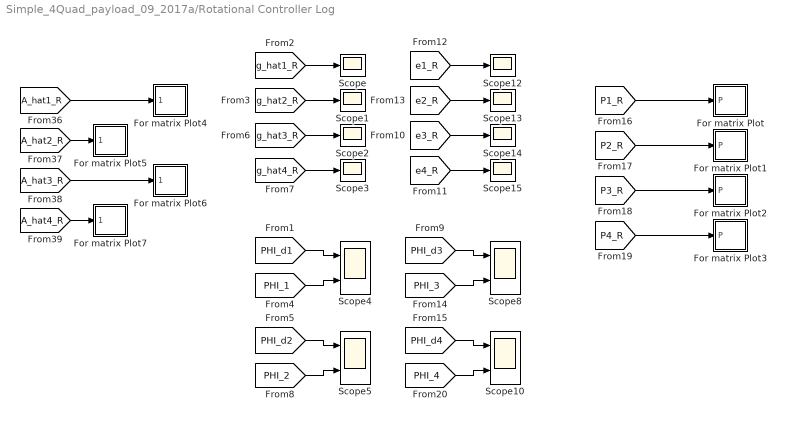
== system Simple_4Quad_payload_09_2017a/Rotational Controller Log ==
  For matrix Plot : Subsystem
  For matrix Plot1 : Subsystem
  For matrix Plot2 : Subsystem
  For matrix Plot3 : Subsystem
  For matrix Plot4 : Subsystem
  For matrix Plot5 : Subsystem
  For matrix Plot6 : Subsystem
  For matrix Plot7 : Subsystem
  Scope{,1..3,12..15} (8 alike) : Scope
  Scope{4..5,8,10} (4 alike) : Scope  NumInputPorts=2
  wires:
  [g_hat1_R] -> Scope/1
  [g_hat3_R] -> Scope2/1
  [g_hat2_R] -> Scope1/1
  [g_hat4_R] -> Scope3/1
  [e2_R] -> Scope13/1
  [P1_R] -> For matrix Plot/1(P)
  [e4_R] -> Scope15/1
  [P4_R] -> For matrix Plot3/1(P)
  [e3_R] -> Scope14/1
  [P3_R] -> For matrix Plot2/1(P)
  [e1_R] -> Scope12/1
  [P2_R] -> For matrix Plot1/1(P)
  [A_hat4_R] -> For matrix Plot7/1(A_hat)
  [A_hat2_R] -> For matrix Plot5/1(A_hat)
  [A_hat1_R] -> For matrix Plot4/1(A_hat)
  [A_hat3_R] -> For matrix Plot6/1(A_hat)
  [PHI_1] -> Scope4/2
  [PHI_d1] -> Scope4/1
  [PHI_d2] -> Scope5/1
  [PHI_2] -> Scope5/2
  [PHI_4] -> Scope10/2
  [PHI_d4] -> Scope10/1
  [PHI_d3] -> Scope8/1
  [PHI_3] -> Scope8/2

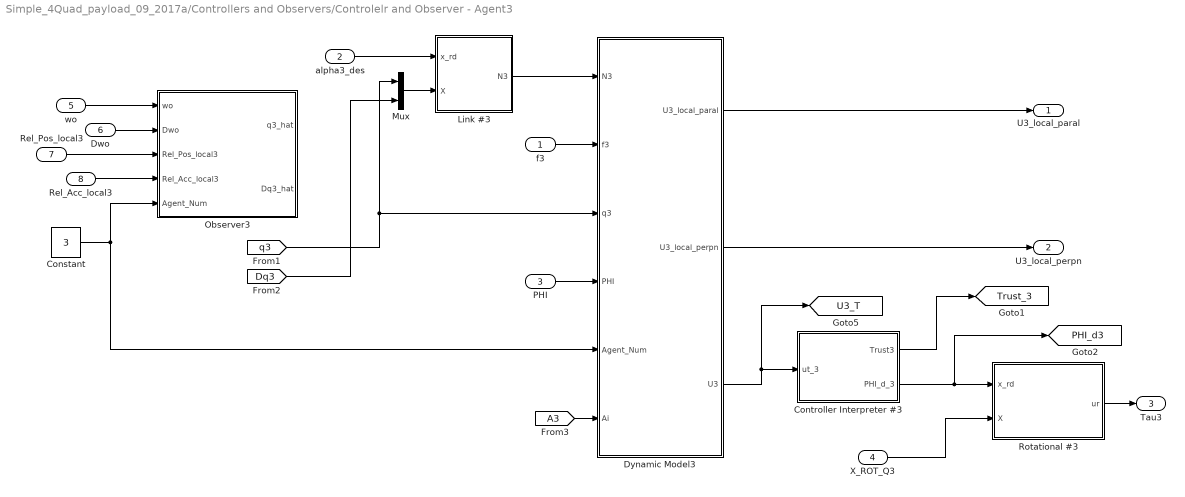
== system Simple_4Quad_payload_09_2017a/Controllers and Observers/Controlelr and Observer - Agent3 ==
  f3 : Inport
  alpha3_des : Inport  Port=2
  PHI : Inport  Port=3
  X_ROT_Q3 : Inport  Port=4
  wo : Inport  Port=5
  Dwo : Inport  Port=6
  Rel_Pos_local3 : Inport  Port=7
  Rel_Acc_local3 : Inport  Port=8
  Constant : Constant  Value=3
  Controller Interpreter #3 : MATLAB Function  TreatAsAtomicUnit=on
  Dynamic Model3 : MATLAB Function  TreatAsAtomicUnit=on
  Link #3 : Subsystem
  Mux : Mux  Inputs=2
  Observer3 : Subsystem
  Rotational #3 : Subsystem
  U3_local_paral : Outport
  U3_local_perpn : Outport  Port=2
  Tau3 : Outport  Port=3
  tag scope: PHI_d3=global, Trust_3=global, U3_T=global
  wires:
  Link #3/1(N3) -> Dynamic Model3/1(N3)
  f3/1 -> Dynamic Model3/2(f3)
  Dynamic Model3/3(U3) -> [U3_T], Controller Interpreter #3/1(ut_3)
  alpha3_des/1 -> Link #3/1(x_rd)
  PHI/1 -> Dynamic Model3/4(PHI)
  Dynamic Model3/1(U3_local_paral) -> U3_local_paral/1
  Controller Interpreter #3/2(PHI_d_3) -> [PHI_d3], Rotational #3/1(x_rd)
  Rotational #3/1(ur) -> Tau3/1
  X_ROT_Q3/1 -> Rotational #3/2(X)
  wo/1 -> Observer3/1(wo)
  Dwo/1 -> Observer3/2(Dwo)
  Rel_Pos_local3/1 -> Observer3/3(Rel_Pos_local3)
  Rel_Acc_local3/1 -> Observer3/4(Rel_Acc_local3)
  Constant/1 -> Dynamic Model3/5(Agent_Num), Observer3/5(Agent_Num)
  [q3] -> Mux/1, Dynamic Model3/3(q3)
  [Dq3] -> Mux/2
  Dynamic Model3/2(U3_local_perpn) -> U3_local_perpn/1
  Controller Interpreter #3/1(Trust3) -> [Trust_3]
  [A3] -> Dynamic Model3/6(Ai)
  Mux/1 -> Link #3/2(X)

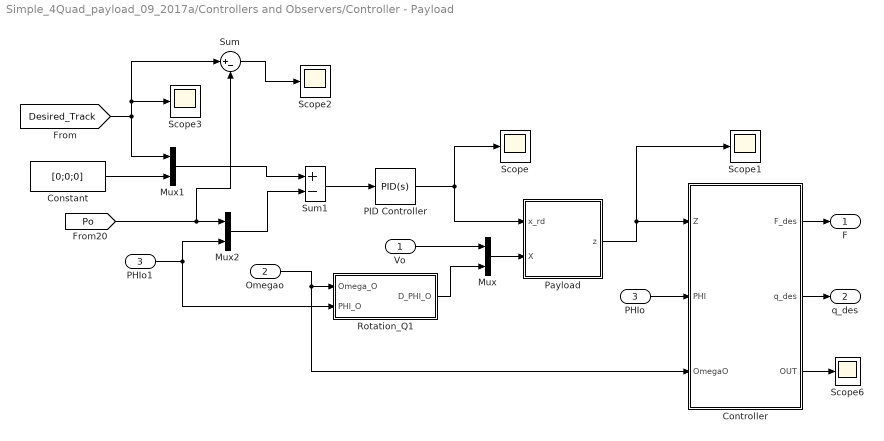
== system Simple_4Quad_payload_09_2017a/Controllers and Observers/Controller - Payload ==
  Vo : Inport
  Omegao : Inport  Port=2
  PHIo : Inport  Port=3
  Constant : Constant  Value=[0;0;0]
  Controller : MATLAB Function  TreatAsAtomicUnit=on
  Mux : Mux  Inputs=2
  Mux1 : Mux  Inputs=2
  Mux2 : Mux  Inputs=2
  PHIo1 : InportShadow  Port=3
  PID Controller : simulink/Continuous/PID Controller  Controller=PID  Form=Parallel  TimeDomain=Continuous-time  SampleTime=-1  IntegratorMethod=Forward Euler  FilterMethod=Forward Euler  ControllerParametersSource=internal  P=1  I=1  D=0  UseFilter=on  N=100  TunerSelectOption=Transfer Function Based (PID Tuner App)  InitialConditionSource=internal  InitialConditionForIntegrator=0  InitialConditionForFilter=0  DifferentiatorICPrevScaledInput=0  ExternalReset=none  TrackingMode=off  Kt=1  LimitOutput=off  UpperSaturationLimit=inf  LowerSaturationLimit=-inf  LinearizeAsGain=on  AntiWindupMode=none  Kb=1  POutMin=[]  POutMax=[]  IOutMin=[]  IOutMax=[]  DOutMin=[]  DOutMax=[]  NOutMin=[]  NOutMax=[]  SumOutMin=[]  SumOutMax=[]  SaturationOutMin=[]  SaturationOutMax=[]  PParamMin=[]  PParamMax=[]  IParamMin=[]  IParamMax=[]  DParamMin=[]  DParamMax=[]  NParamMin=[]  NParamMax=[]  KbParamMin=[]  KbParamMax=[]  KtParamMin=[]  KtParamMax=[]  KbOutMin=[]  KbOutMax=[]  KtOutMin=[]  KtOutMax=[]  IntegratorOutMin=[]  IntegratorOutMax=[]  FilterOutMin=[]  FilterOutMax=[]  SumI1OutMin=[]  SumI1OutMax=[]  SumI2OutMin=[]  SumI2OutMax=[]  SumI3OutMin=[]  SumI3OutMax=[]  SumI4OutMin=[]  SumI4OutMax=[]  SumDOutMin=[]  SumDOutMax=[]  DifferentiatorOutMin=[]  DifferentiatorOutMax=[]  FilterDiffOutCoefMin=[]  FilterDiffOutCoefMax=[]  ReciprocalOutMin=[]  ReciprocalOutMax=[]  SumDenOutMin=[]  SumDenOutMax=[]  SumNumOutMin=[]  SumNumOutMax=[]  DivideOutMin=[]  DivideOutMax=[]  IntegratorContinuousStateAttributes=''  IntegratorStateMustResolveToSignalObject=off  IntegratorRTWStateStorageClass=Auto  FilterContinuousStateAttributes=''  FilterStateMustResolveToSignalObject=off  FilterRTWStateStorageClass=Auto  ParallelPVariant=InternalParameters  IdealPVariant=Disabled  IVariant=InternalParameters  DVariant=InternalParameters  IntegratorVariant=Continuous  SatVariant=Disabled  AWVariant=Passthrough  PCopyVariant=Disabled  TRVariant=Disabled  FdbkBlocksVariant=Forward  IdealPFdbkVariant=Disabled  SatFdbkVariant=Disabled  DerivativeFilterVariant=ContFilter  NVariant=InternalParameters  NCopyVariant=Disabled  FilterICVariant=InternalICsFilter  IntegratorICVariant=InternalICs  ExternalResetVariant=Disabled  TRSumVariant=Passthrough  SumFdbkVariant=Disabled  SumVariant=Sum_PID
  Payload : Subsystem
  Rotation_Q1 : Subsystem
  Scope{,1..3,6} (5 alike) : Scope
  Sum : Sum  Inputs=|+-
  Sum1 : Sum  Inputs=+-
  F : Outport
  q_des : Outport  Port=2
  wires:
  Controller/3(OUT) -> Scope6/1
  Controller/2(q_des) -> q_des/1
  Controller/1(F_des) -> F/1
  PHIo/1 -> Controller/2(PHI)
  Payload/1(z) -> Scope1/1, Controller/1(Z)
  Mux/1 -> Payload/2(X)
  Vo/1 -> Mux/1
  Rotation_Q1/1(D_PHI_O) -> Mux/2
  [Desired_Track] -> Scope3/1, Sum/1, Mux1/1
  Constant/1 -> Mux1/2
  Mux2/1 -> Sum1/2
  PHIo1/1 -> Rotation_Q1/2(PHI_O), Mux2/2
  [Po] -> Sum/2, Mux2/1
  Omegao/1 -> Controller/3(OmegaO), Rotation_Q1/1(Omega_O)
  Sum/1 -> Scope2/1
  Mux1/1 -> Sum1/1
  Sum1/1 -> PID Controller/1
  PID Controller/1 -> Payload/1(x_rd), Scope/1

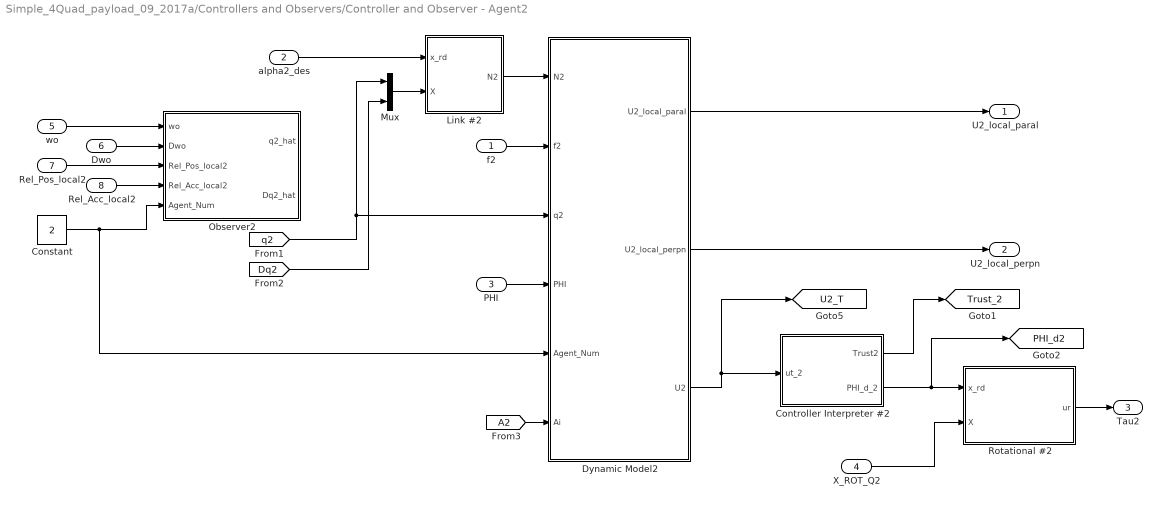
== system Simple_4Quad_payload_09_2017a/Controllers and Observers/Controller and Observer - Agent2 ==
  f2 : Inport
  alpha2_des : Inport  Port=2
  PHI : Inport  Port=3
  X_ROT_Q2 : Inport  Port=4
  wo : Inport  Port=5
  Dwo : Inport  Port=6
  Rel_Pos_local2 : Inport  Port=7
  Rel_Acc_local2 : Inport  Port=8
  Constant : Constant  Value=2
  Controller Interpreter #2 : MATLAB Function  TreatAsAtomicUnit=on
  Dynamic Model2 : MATLAB Function  TreatAsAtomicUnit=on
  Link #2 : Subsystem
  Mux : Mux  Inputs=2
  Observer2 : Subsystem
  Rotational #2 : Subsystem
  U2_local_paral : Outport
  U2_local_perpn : Outport  Port=2
  Tau2 : Outport  Port=3
  tag scope: PHI_d2=global, Trust_2=global, U2_T=global
  wires:
  Dynamic Model2/3(U2) -> Controller Interpreter #2/1(ut_2), [U2_T]
  alpha2_des/1 -> Link #2/1(x_rd)
  f2/1 -> Dynamic Model2/2(f2)
  PHI/1 -> Dynamic Model2/4(PHI)
  Link #2/1(N2) -> Dynamic Model2/1(N2)
  Dynamic Model2/1(U2_local_paral) -> U2_local_paral/1
  Controller Interpreter #2/2(PHI_d_2) -> [PHI_d2], Rotational #2/1(x_rd)
  Rotational #2/1(ur) -> Tau2/1
  X_ROT_Q2/1 -> Rotational #2/2(X)
  wo/1 -> Observer2/1(wo)
  Dwo/1 -> Observer2/2(Dwo)
  Rel_Pos_local2/1 -> Observer2/3(Rel_Pos_local2)
  Rel_Acc_local2/1 -> Observer2/4(Rel_Acc_local2)
  Constant/1 -> Observer2/5(Agent_Num), Dynamic Model2/5(Agent_Num)
  [q2] -> Mux/1, Dynamic Model2/3(q2)
  [Dq2] -> Mux/2
  Dynamic Model2/2(U2_local_perpn) -> U2_local_perpn/1
  Controller Interpreter #2/1(Trust2) -> [Trust_2]
  [A2] -> Dynamic Model2/6(Ai)
  Mux/1 -> Link #2/2(X)

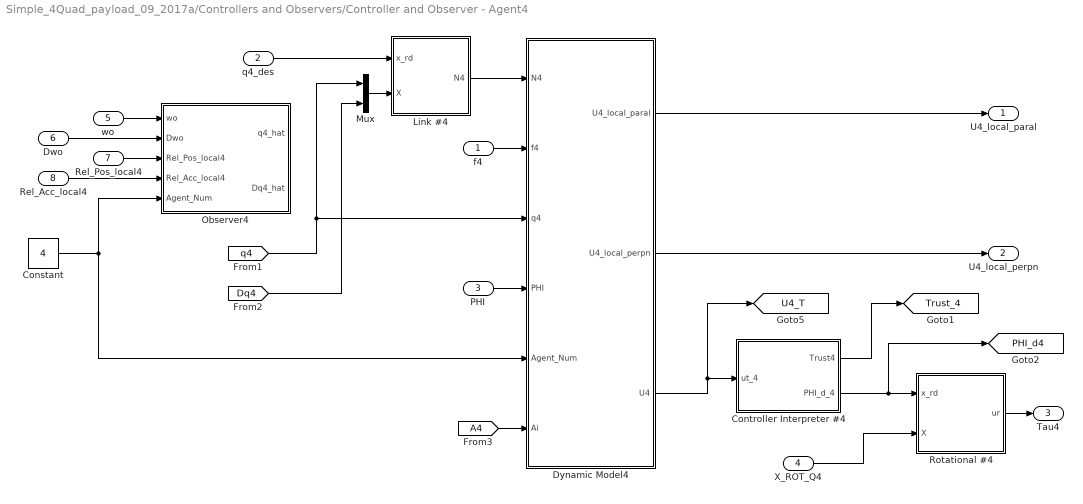
== system Simple_4Quad_payload_09_2017a/Controllers and Observers/Controller and Observer - Agent4 ==
  f4 : Inport
  q4_des : Inport  Port=2
  PHI : Inport  Port=3
  X_ROT_Q4 : Inport  Port=4
  wo : Inport  Port=5
  Dwo : Inport  Port=6
  Rel_Pos_local4 : Inport  Port=7
  Rel_Acc_local4 : Inport  Port=8
  Constant : Constant  Value=4
  Controller Interpreter #4 : MATLAB Function  TreatAsAtomicUnit=on
  Dynamic Model4 : MATLAB Function  TreatAsAtomicUnit=on
  Link #4 : Subsystem
  Mux : Mux  Inputs=2
  Observer4 : Subsystem
  Rotational #4 : Subsystem
  U4_local_paral : Outport
  U4_local_perpn : Outport  Port=2
  Tau4 : Outport  Port=3
  tag scope: PHI_d4=global, Trust_4=global, U4_T=global
  wires:
  Dynamic Model4/3(U4) -> Controller Interpreter #4/1(ut_4), [U4_T]
  Link #4/1(N4) -> Dynamic Model4/1(N4)
  PHI/1 -> Dynamic Model4/4(PHI)
  f4/1 -> Dynamic Model4/2(f4)
  q4_des/1 -> Link #4/1(x_rd)
  Dynamic Model4/1(U4_local_paral) -> U4_local_paral/1
  Controller Interpreter #4/2(PHI_d_4) -> [PHI_d4], Rotational #4/1(x_rd)
  Rotational #4/1(ur) -> Tau4/1
  Rel_Pos_local4/1 -> Observer4/3(Rel_Pos_local4)
  Dwo/1 -> Observer4/2(Dwo)
  wo/1 -> Observer4/1(wo)
  Rel_Acc_local4/1 -> Observer4/4(Rel_Acc_local4)
  Constant/1 -> Observer4/5(Agent_Num), Dynamic Model4/5(Agent_Num)
  [q4] -> Mux/1, Dynamic Model4/3(q4)
  [Dq4] -> Mux/2
  Dynamic Model4/2(U4_local_perpn) -> U4_local_perpn/1
  X_ROT_Q4/1 -> Rotational #4/2(X)
  Controller Interpreter #4/1(Trust4) -> [Trust_4]
  [A4] -> Dynamic Model4/6(Ai)
  Mux/1 -> Link #4/2(X)
